simulink model "DC_Motor_OpenLoop"  (R2025b)
settings: Solver=VariableStepAuto  StartTime=0.0  StopTime=5  RelTol=1e-3

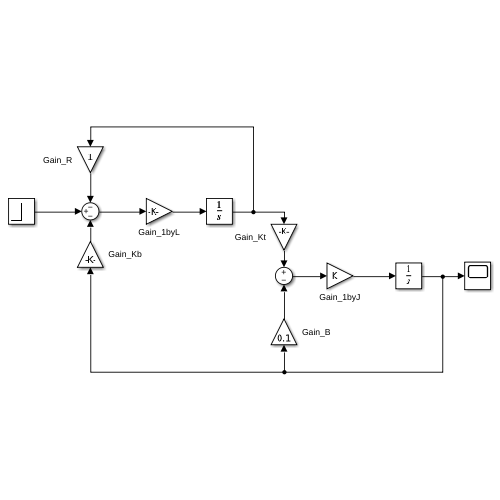
[thumbnail: Simulink's stored preview of the top-level diagram]
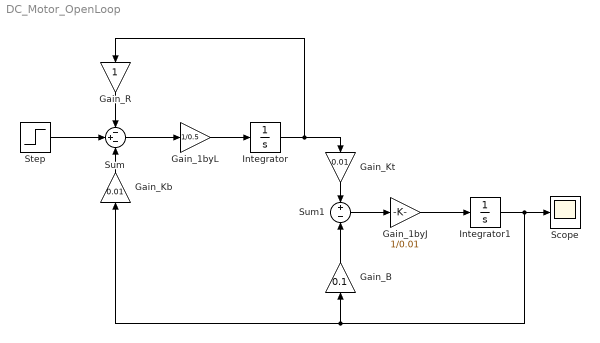
== system DC_Motor_OpenLoop ==
  Gain_1byJ : Gain  Gain=1/0.01
  Gain_1byL : Gain  Gain=1/0.5
  Gain_B : Gain  Gain=0.1
  Gain_Kb : Gain  Gain=0.01
  Gain_Kt : Gain  Gain=0.01
  Gain_R : Gain  Tag=Gain_R
  Integrator : Integrator
  Integrator1 : Integrator
  Scope : Scope
  Step : Step  After=12  SampleTime=0
  Sum : Sum  Inputs=-+-
  Sum1 : Sum  Inputs=+-
  wires:
  Gain_1byJ/1 -> Integrator1/1
  Sum1/1 -> Gain_1byJ/1
  Step/1 -> Sum/2
  Sum/1 -> Gain_1byL/1
  Gain_1byL/1 -> Integrator/1
  Gain_Kt/1 -> Sum1/1
  Gain_B/1 -> Sum1/2
  Integrator/1 -> Gain_Kt/1, Gain_R/1
  Gain_R/1 -> Sum/1
  Integrator1/1 -> Scope/1, Gain_B/1, Gain_Kb/1
  Gain_Kb/1 -> Sum/3
